simulink model "quarter_car_suspension"  (R2024b)
settings: Solver=VariableStepAuto  StartTime=0.0  StopTime=20  RelTol=1e-3
InitFcn:
  | mb=320;
  | mw=40;
  | Cs=1800;
  | kt=200000;
  | ks=20000;
  | v=36;
libraries: simulink x4
settings Model: Creator=Y1509  LastModifiedBy=Y1509

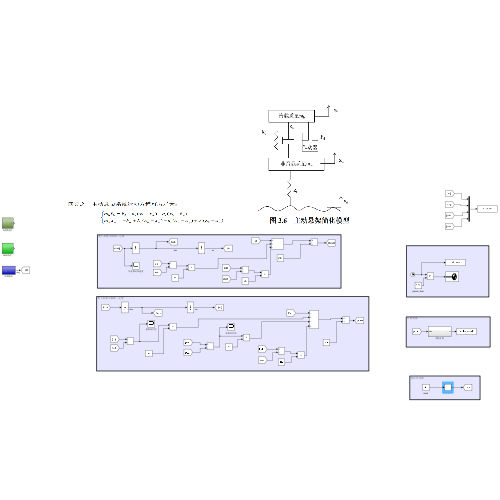
[thumbnail: Simulink's stored preview of the top-level diagram]
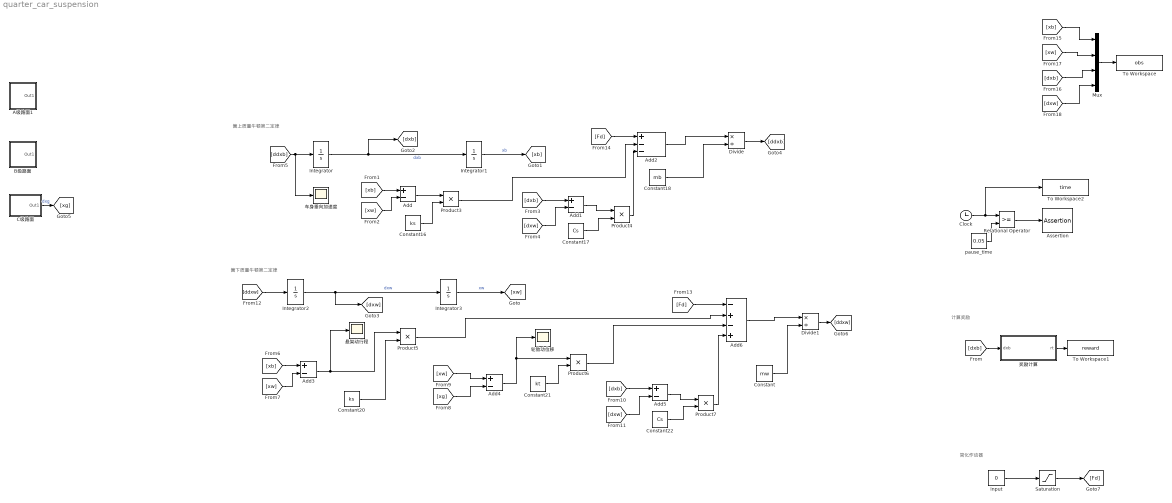
== system quarter_car_suspension ==
  note: 简化作动器
  note: 计算奖励
  note: 簧下质量牛顿第二定律
  note: 簧上质量牛顿第二定律
  Add{,1,3..5} (5 alike) : Sum  Inputs=+-
  Add2 : Sum  Inputs=+--
  Add6 : Sum  Inputs=-+-+
  Assertion : Assertion  AssertionFailFcn=set_param(bdroot,'SimulationCommand','pause')  StopWhenAssertionFail=off
  A级路面1 : Subsystem
  B级路面 : Subsystem
  Clock : Clock
  Constant : Constant  Value=mw
  Constant16 : Constant  Value=ks
  Constant17 : Constant  Value=Cs
  Constant18 : Constant  Value=mb
  Constant20 : Constant  Value=ks
  Constant21 : Constant  Value=kt
  Constant22 : Constant  Value=Cs
  C级路面 : Subsystem
  Divide : Product  Inputs=*/
  Divide1 : Product  Inputs=*/
  Integrator{,1..3} (4 alike) : Integrator
  Mux : Mux
  Product{3..7} (5 alike) : Product
  Relational Operator : RelationalOperator  OutDataTypeStr=boolean  RndMeth=Simplest  InputSameDT=off
  Saturation : Saturate  UpperLimit=1500  LowerLimit=-1500
  To Workspace : ToWorkspace  VariableName=obs  SampleTime=-1
  To Workspace1 : ToWorkspace  VariableName=reward  SampleTime=-1
  To Workspace2 : ToWorkspace  VariableName=time  SampleTime=-1
  input : Constant  Value=0
  pause_time : Constant  Value=0.05
  奖励计算 : Subsystem
  悬架动行程 : Scope
  车身垂向加速度 : Scope
  轮胎动位移 : Scope
  wires:
  Integrator/1 -> [dxb], Integrator1/1  "dxb"
  Integrator1/1 -> [xb]  "xb"
  Integrator2/1 -> [dxw], Integrator3/1  "dxw"
  Integrator3/1 -> [xw]  "xw"
  [xb] -> Add/1
  [xw] -> Add/2
  Add/1 -> Product3/1
  Constant16/1 -> Product3/2
  [dxb] -> Add1/1
  [dxw] -> Add1/2
  Add1/1 -> Product4/1
  Constant17/1 -> Product4/2
  [Fd] -> Add2/1
  Product3/1 -> Add2/2
  Product4/1 -> Add2/3
  Add2/1 -> Divide/1
  Constant18/1 -> Divide/2
  Divide/1 -> [ddxb]
  [ddxb] -> 车身垂向加速度/1, Integrator/1
  Constant20/1 -> Product5/2
  Add3/1 -> 悬架动行程/1, Product5/1
  [xw] -> Add3/2
  [xb] -> Add3/1
  [xw] -> Add4/1
  [xg] -> Add4/2
  Add4/1 -> 轮胎动位移/1, Product6/1
  Constant21/1 -> Product6/2
  Constant22/1 -> Product7/2
  Add5/1 -> Product7/1
  [dxw] -> Add5/2
  [dxb] -> Add5/1
  [Fd] -> Add6/1
  Product5/1 -> Add6/2
  Product6/1 -> Add6/3
  Product7/1 -> Add6/4
  [ddxw] -> Integrator2/1
  Constant/1 -> Divide1/2
  Divide1/1 -> [ddxw]
  Add6/1 -> Divide1/1
  C级路面/1(Out1) -> [xg]  "dxg"
  [dxb] -> 奖励计算/1(dxb)
  Clock/1 -> To Workspace2/1, Relational Operator/1
  pause_time/1 -> Relational Operator/2
  Relational Operator/1 -> Assertion/1
  [xb] -> Mux/1
  [xw] -> Mux/2
  [dxb] -> Mux/3
  [dxw] -> Mux/4
  Mux/1 -> To Workspace/1
  奖励计算/1(rt) -> To Workspace1/1
  input/1 -> Saturation/1
  Saturation/1 -> [Fd]

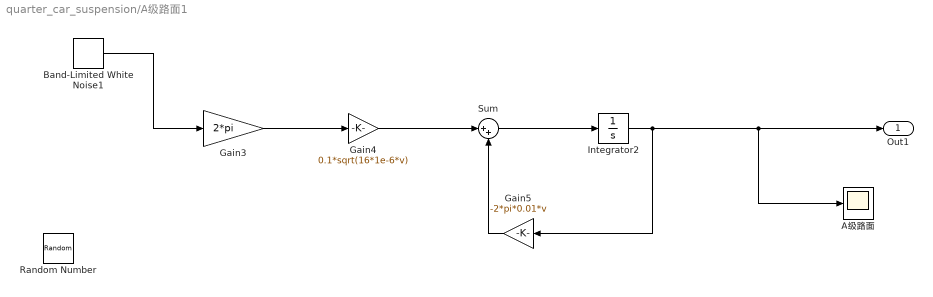
== system quarter_car_suspension/A级路面1 ==
  A级路面 : Scope
  Band-Limited White Noise1 : simulink/Sources/Band-Limited White Noise  Cov=[0.4]  Ts=0.01  seed=233
  Gain3 : Gain  Gain=2*pi
  Gain4 : Gain  Gain=0.1*sqrt(16*1e-6*v)
  Gain5 : Gain  Gain=-2*pi*0.01*v
  Integrator2 : Integrator
  Random Number : RandomNumber  Seed=233  SampleTime=0.1
  Sum : Sum  Inputs=|++
  Out1 : Outport
  wires:
  Band-Limited White Noise1/1 -> Gain3/1
  Gain3/1 -> Gain4/1
  Gain4/1 -> Sum/1
  Gain5/1 -> Sum/2
  Integrator2/1 -> Gain5/1, Out1/1, A级路面/1
  Sum/1 -> Integrator2/1

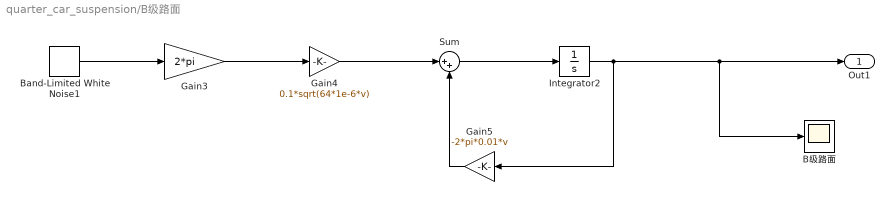
== system quarter_car_suspension/B级路面 ==
  Band-Limited White Noise1 : simulink/Sources/Band-Limited White Noise  Cov=[0.4]  Ts=0.01  seed=233
  B级路面 : Scope
  Gain3 : Gain  Gain=2*pi
  Gain4 : Gain  Gain=0.1*sqrt(64*1e-6*v)
  Gain5 : Gain  Gain=-2*pi*0.01*v
  Integrator2 : Integrator
  Sum : Sum  Inputs=|++
  Out1 : Outport
  wires:
  Sum/1 -> Integrator2/1
  Integrator2/1 -> B级路面/1, Out1/1, Gain5/1
  Gain5/1 -> Sum/2
  Gain4/1 -> Sum/1
  Gain3/1 -> Gain4/1
  Band-Limited White Noise1/1 -> Gain3/1

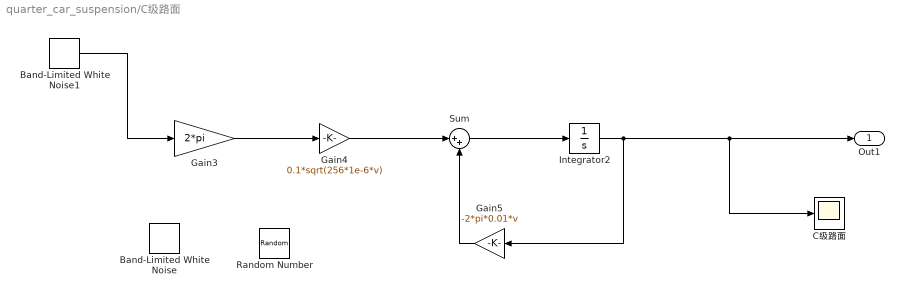
== system quarter_car_suspension/C级路面 ==
  Band-Limited White Noise : simulink/Sources/Band-Limited White Noise  Cov=[0.1]  Ts=0.1  seed=[23341]
  Band-Limited White Noise1 : simulink/Sources/Band-Limited White Noise  Cov=[0.4]  Ts=0.01  seed=[23341]
  C级路面 : Scope
  Gain3 : Gain  Gain=2*pi
  Gain4 : Gain  Gain=0.1*sqrt(256*1e-6*v)
  Gain5 : Gain  Gain=-2*pi*0.01*v
  Integrator2 : Integrator
  Random Number : RandomNumber  SampleTime=0.1
  Sum : Sum  Inputs=|++
  Out1 : Outport
  wires:
  Gain3/1 -> Gain4/1
  Gain4/1 -> Sum/1
  Gain5/1 -> Sum/2
  Integrator2/1 -> Gain5/1, Out1/1, C级路面/1
  Sum/1 -> Integrator2/1
  Band-Limited White Noise1/1 -> Gain3/1

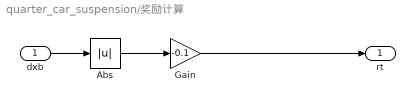
== system quarter_car_suspension/奖励计算 ==
  dxb : Inport
  Abs : Abs  SaturateOnIntegerOverflow=off
  Gain : Gain  Gain=-0.1
  rt : Outport
  wires:
  dxb/1 -> Abs/1
  Abs/1 -> Gain/1
  Gain/1 -> rt/1
